simulink model "SMC"  (R2018a)
settings: Solver=VariableStepAuto  StartTime=0.0  StopTime=15  RelTol=1e-3
settings Model: Creator=Administrator  LastModifiedBy=Administrator

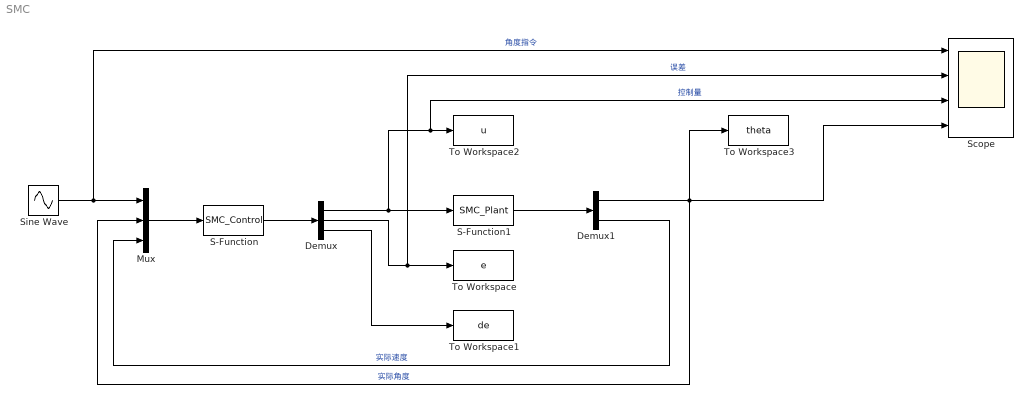
== system SMC ==
  Demux : Demux  Outputs=3
  Demux1 : Demux  Outputs=2
  Mux : Mux  Inputs=3
  S-Function : S-Function  FunctionName=SMC_Control  SFunctionDeploymentMode=off  EnableBusSupport=off
  S-Function1 : S-Function  FunctionName=SMC_Plant  SFunctionDeploymentMode=off  EnableBusSupport=off
  Scope : Scope  NumInputPorts=4
  Sine Wave : Sin  SampleTime=0
  To Workspace : ToWorkspace  VariableName=e  SampleTime=-1
  To Workspace1 : ToWorkspace  VariableName=de  SampleTime=-1
  To Workspace2 : ToWorkspace  VariableName=u  SampleTime=-1
  To Workspace3 : ToWorkspace  VariableName=theta  SampleTime=-1
  wires:
  Mux/1 -> S-Function/1
  S-Function/1 -> Demux/1
  Demux/1 -> Scope/3, To Workspace2/1, S-Function1/1  "控制量"
  Demux/2 -> Scope/2, To Workspace/1  "误差"
  Demux/3 -> To Workspace1/1
  S-Function1/1 -> Demux1/1
  Sine Wave/1 -> Scope/1, Mux/1  "角度指令"
  Demux1/1 -> Scope/4, To Workspace3/1, Mux/2  "实际角度"
  Demux1/2 -> Mux/3  "实际速度"
